simulink model "control_system_model_template"  (R2022b)
settings: Solver=VariableStepAuto  StartTime=0.0  StopTime=10.0  RelTol=1e-3
libraries: SignalEditorBlockLib x1
settings Model: DataDictionary=control_system_data.sldd  Creator=tshintai  LastModifiedBy=tshintai
settings DebuggingCC: UnconnectedInputMsg=warning  UnconnectedOutputMsg=warning  UnconnectedLineMsg=warning
settings ModelReferenceCC: EnableRefExpFcnMdlSchedulingChecks=on
settings RTWCC: DLArmComputeVersion=19.05

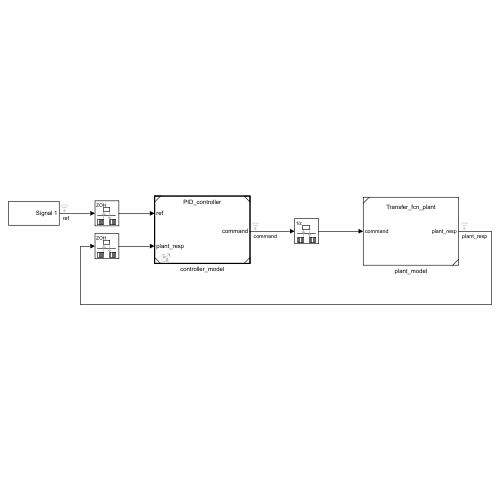
[thumbnail: Simulink's stored preview of the top-level diagram]
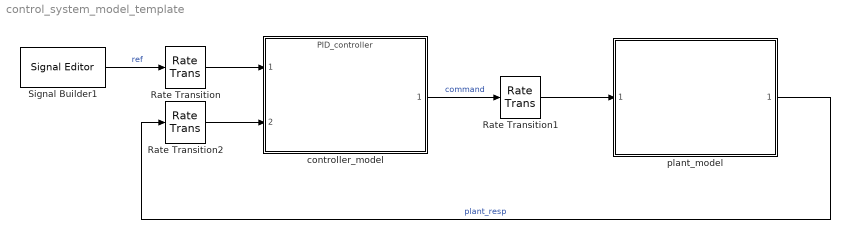
== system control_system_model_template ==
  Rate Transition : RateTransition  OutPortSampleTime=ts
  Rate Transition1 : RateTransition
  Rate Transition2 : RateTransition  OutPortSampleTime=ts
  Signal Builder1 : SignalEditorBlockLib/Signal Editor  FileName=control_system_ref_signal.mat  ActiveScenario=Group_1  ActiveSignal=Signal 1  IsBus=off  OutputBusObjectStr=Bus: BusObject  SampleTime=0  OutputAfterFinalValue=Holding final value  Unit=inherit  PreserveSignalName=on
  controller_model : ModelReference  ModelNameDialog=PID_controller  SimulationMode=Normal  ModelReferenceVersion=4.0
  plant_model : Subsystem  ReferencedSubsystem=Transfer_fcn_plant
  wires:
  Signal Builder1/1 -> Rate Transition/1  "ref"
  Rate Transition/1 -> controller_model/1
  controller_model/1 -> Rate Transition1/1  "command"
  Rate Transition2/1 -> controller_model/2
  Rate Transition1/1 -> plant_model/1
  plant_model/1 -> Rate Transition2/1  "plant_resp"
